simulink model "adaptive_normalised_mit_rule"  (R2015b)
settings: Solver=VariableStepAuto  StartTime=0.0  StopTime=100  RelTol=1e-3
settings Model: Creator=santhosh  LastModifiedBy=uchiha

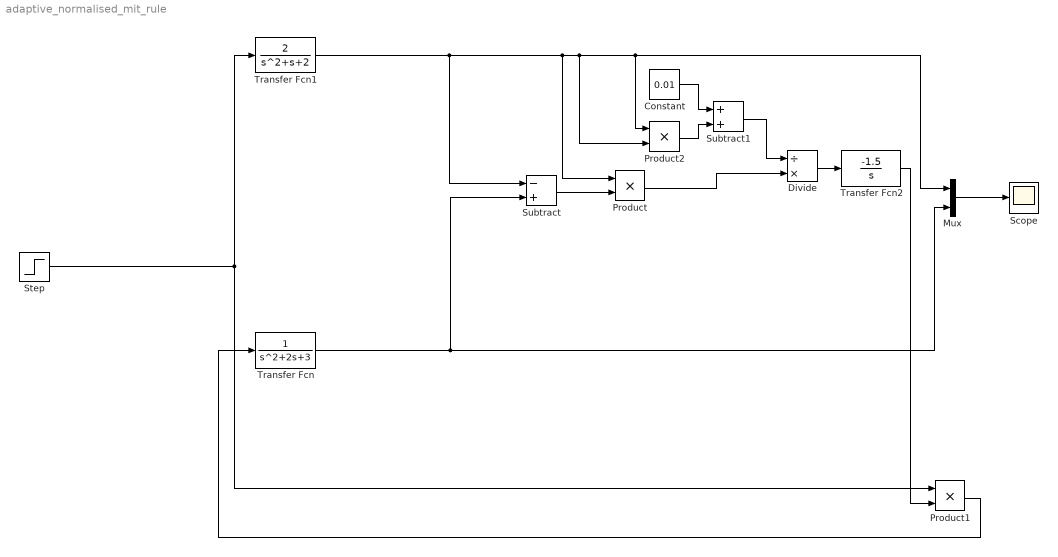
== system adaptive_normalised_mit_rule ==
  Constant : Constant  Value=0.01
  Divide : Product  Inputs=/*
  Mux : Mux  Inputs=2
  Product : Product
  Product1 : Product
  Product2 : Product
  Scope : Scope
  Step : Step  After=4  SampleTime=0
  Subtract : Sum  Inputs=-+
  Subtract1 : Sum
  Transfer Fcn : TransferFcn  Denominator=[1 2 3]
  Transfer Fcn1 : TransferFcn  Numerator=[2]  Denominator=[1 1 2]  ContinuousStateAttributes='reference'
  Transfer Fcn2 : TransferFcn  Numerator=[-1.5]  Denominator=[1 0]
  wires:
  Subtract/1 -> Product/2
  Transfer Fcn2/1 -> Product1/2
  Product1/1 -> Transfer Fcn/1
  Mux/1 -> Scope/1
  Transfer Fcn1/1 -> Subtract/1, Product/1, Product2/2, Product2/1, Mux/1
  Product2/1 -> Subtract1/2
  Constant/1 -> Subtract1/1
  Divide/1 -> Transfer Fcn2/1
  Subtract1/1 -> Divide/1
  Product/1 -> Divide/2
  Step/1 -> Product1/1, Transfer Fcn1/1
  Transfer Fcn/1 -> Subtract/2, Mux/2
